simulink model "FirstOrderSystem"  (R2023b)
settings: Solver=VariableStepAuto  StartTime=0.0  StopTime=10.0  RelTol=1e-3
values from neighbouring files (symbols this model uses):
  G_den3 = [M B k]    [TransferFunction.m]
  G_num3 = [1]    [TransferFunction.m]
settings Model: Creator=Emanuel  LastModifiedBy=Emanuel

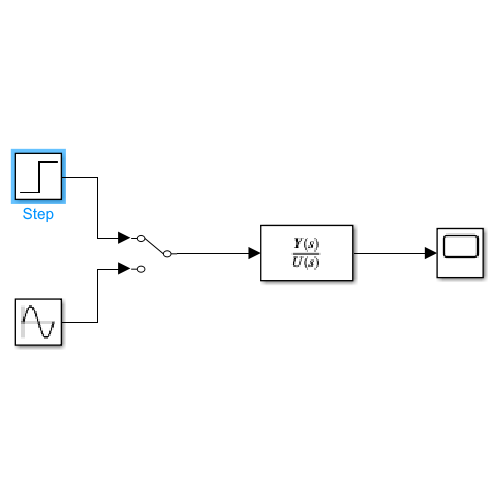
[thumbnail: Simulink's stored preview of the top-level diagram]
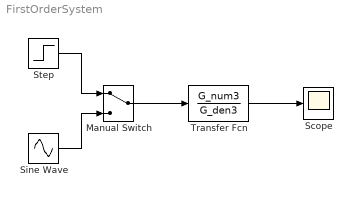
== system FirstOrderSystem ==
  Manual Switch : ManualSwitch
  Scope : Scope
  Sine Wave : Sin  SampleTime=0
  Step : Step  Time=0  SampleTime=0
  Transfer Fcn : TransferFcn  Numerator=G_num3  Denominator=G_den3
  wires:
  Transfer Fcn/1 -> Scope/1
  Manual Switch/1 -> Transfer Fcn/1
  Step/1 -> Manual Switch/1
  Sine Wave/1 -> Manual Switch/2
